simulink model "ahrs_wrk"  (R2021b)
settings: Solver=ode1be  StartTime=0.0  StopTime=tsc.Time(end)  FixedStep=0.01  RelTol=1e-3
values from neighbouring files (symbols this model uses):
  tsc = flatball_6dof_post( simout.logsout, disc, amb)    [flatball_6dof_wrk.m]    (also in hummel_thesis_mdl_validation.m = flatball_6dof_post( logsout, disc, amb))
libraries: mspfiltlib x1
settings Model: Creator=schae  LastModifiedBy=schae

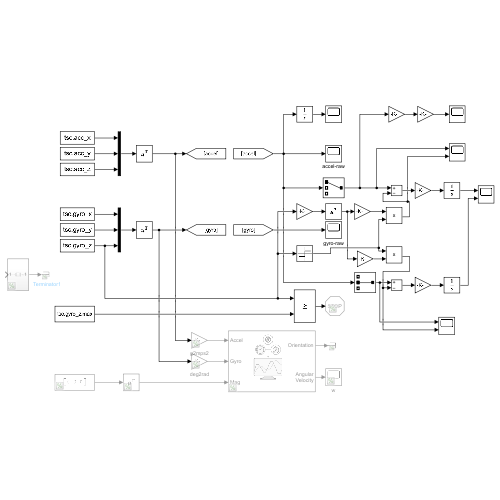
[thumbnail: Simulink's stored preview of the top-level diagram]
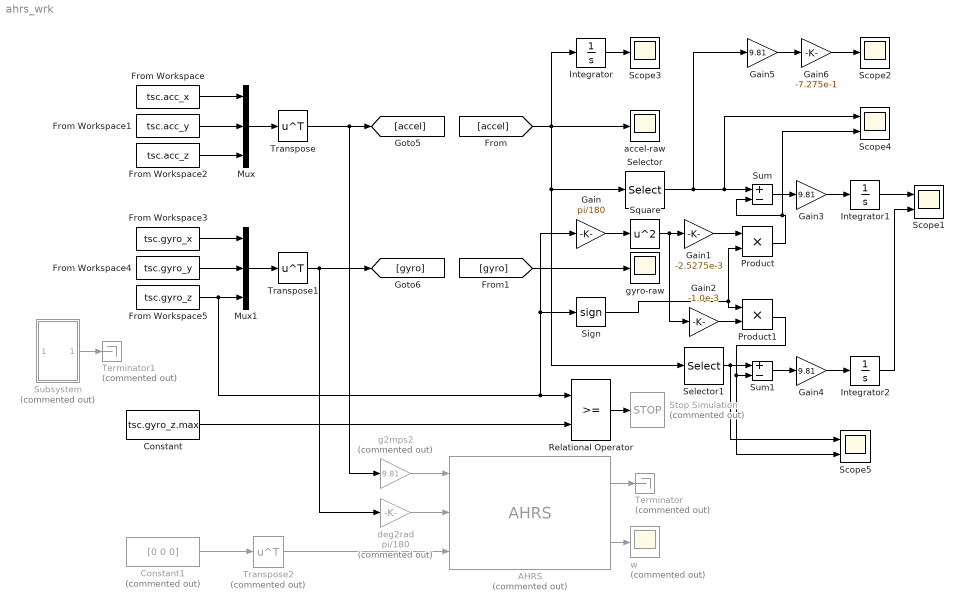
== system ahrs_wrk ==
  AHRS : mspfiltlib/AHRS  Commented=on  DispRefFrame=ENU  DecimationFactor=1  InitialProcessNoise=ahrsfilter.defaultProcessNoise  OrientationFormat=Rotation matrix  SimulateUsing=Interpreted execution  AccelerometerNoise=0.0001924722  GyroscopeNoise=9.1385e-5  MagnetometerNoise=0.1  GyroscopeDriftNoise=3.0462e-13  LinearAccelerationNoise=0.0096236100000000012  MagneticDisturbanceNoise=0.5  LinearAccelerationDecayFactor=0.5  MagneticDisturbanceDecayFactor=0.5  ExpectedMagneticFieldStrength=50
      settings: SourceProductBaseCode=TF,NV
  Constant : Constant  Value=tsc.gyro_z.max
  Constant1 : Constant  Commented=on  Value=[0 0 0]
  From Workspace : FromWorkspace  VariableName=tsc.acc_x  SampleTime=0.01  OutputAfterFinalValue=Holding final value
  From Workspace1 : FromWorkspace  VariableName=tsc.acc_y  SampleTime=0.01  OutputAfterFinalValue=Holding final value
  From Workspace2 : FromWorkspace  VariableName=tsc.acc_z  SampleTime=0.01  OutputAfterFinalValue=Holding final value
  From Workspace3 : FromWorkspace  VariableName=tsc.gyro_x  SampleTime=0.01  OutputAfterFinalValue=Holding final value
  From Workspace4 : FromWorkspace  VariableName=tsc.gyro_y  SampleTime=0.01  OutputAfterFinalValue=Holding final value
  From Workspace5 : FromWorkspace  VariableName=tsc.gyro_z  SampleTime=0.01  OutputAfterFinalValue=Holding final value
  Gain : Gain  Gain=pi/180
  Gain1 : Gain  Gain=-2.5275e-3
  Gain2 : Gain  Gain=-1.0e-3
  Gain3 : Gain  Gain=9.81
  Gain4 : Gain  Gain=9.81
  Gain5 : Gain  Gain=9.81
  Gain6 : Gain  Gain=-7.275e-1
  Integrator : Integrator
  Integrator1 : Integrator
  Integrator2 : Integrator
  Mux : Mux  Inputs=3
  Mux1 : Mux  Inputs=3
  Product : Product
  Product1 : Product
  Relational Operator : RelationalOperator  OutDataTypeStr=boolean  RndMeth=Simplest
  Scope1 : Scope  NumInputPorts=2
  Scope2 : Scope
  Scope3 : Scope
  Scope4 : Scope  NumInputPorts=2
  Scope5 : Scope  NumInputPorts=2
  Selector : Selector  InputPortWidth=3  IndexOptions=Index vector (dialog)  Indices=[1]  OutputSizes=1
  Selector1 : Selector  InputPortWidth=3  IndexOptions=Index vector (dialog)  Indices=[2]  OutputSizes=1
  Sign : Signum
  Square : Math  Operator=square  SaturateOnIntegerOverflow=on
  Stop Simulation : Stop  Commented=on
  Subsystem : Subsystem  Commented=on
  Sum : Sum  Inputs=+-
  Sum1 : Sum  Inputs=+-
  Terminator : Terminator  Commented=on
  Terminator1 : Terminator  Commented=on
  Transpose : Math  Operator=transpose  SaturateOnIntegerOverflow=on
  Transpose1 : Math  Operator=transpose  SaturateOnIntegerOverflow=on
  Transpose2 : Math  Commented=on  Operator=transpose  SaturateOnIntegerOverflow=on
  accel-raw : Scope
  deg2rad : Gain  Commented=on  Gain=pi/180
  g2mps2 : Gain  Commented=on  Gain=9.81
  gyro-raw : Scope
  w : Scope  Commented=on
  wires:
  From Workspace2/1 -> Mux/3
  From Workspace1/1 -> Mux/2
  From Workspace3/1 -> Mux1/1
  Mux/1 -> Transpose/1
  From Workspace/1 -> Mux/1
  From Workspace5/1 -> Sign/1, Gain/1, Relational Operator/1, Mux1/3
  Mux1/1 -> Transpose1/1
  From Workspace4/1 -> Mux1/2
  [gyro] -> gyro-raw/1
  Integrator/1 -> Scope3/1
  Constant/1 -> Relational Operator/2
  Relational Operator/1 -> Stop Simulation/1
  Constant1/1 -> Transpose2/1
  AHRS/2 -> w/1
  Transpose/1 -> g2mps2/1, [accel]
  Transpose1/1 -> deg2rad/1, [gyro]
  Transpose2/1 -> AHRS/3
  g2mps2/1 -> AHRS/1
  deg2rad/1 -> AHRS/2
  AHRS/1 -> Terminator/1
  Subsystem/1(Out1) -> Terminator1/1
  Selector/1 -> Gain5/1, Scope4/1, Sum/1
  Gain/1 -> Square/1
  Square/1 -> Gain2/1, Gain1/1
  Selector1/1 -> Sum1/1, Scope5/1
  Integrator1/1 -> Scope1/1
  Sum/1 -> Gain3/1
  Sum1/1 -> Gain4/1
  Integrator2/1 -> Scope1/2
  [accel] -> Selector/1, Selector1/1, Integrator/1, accel-raw/1
  Gain3/1 -> Integrator1/1
  Gain4/1 -> Integrator2/1
  Gain5/1 -> Gain6/1
  Gain6/1 -> Scope2/1
  Gain1/1 -> Product/1
  Sign/1 -> Product1/1, Product/2
  Product/1 -> Scope4/2, Sum/2
  Gain2/1 -> Product1/2
  Product1/1 -> Scope5/2, Sum1/2

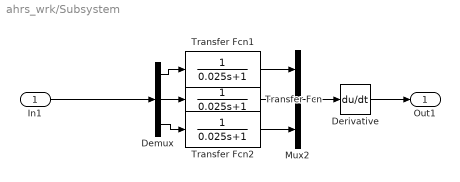
== system ahrs_wrk/Subsystem ==
  In1 : Inport
  Demux : Demux  Outputs=3
  Derivative : Derivative
  Mux2 : Mux  Inputs=3
  Transfer Fcn : TransferFcn  Denominator=[0.025 1]
  Transfer Fcn1 : TransferFcn  Denominator=[0.025 1]
  Transfer Fcn2 : TransferFcn  Denominator=[0.025 1]
  Out1 : Outport
  wires:
  Transfer Fcn/1 -> Mux2/2
  Demux/1 -> Transfer Fcn1/1
  Mux2/1 -> Derivative/1
  Demux/2 -> Transfer Fcn/1
  Transfer Fcn1/1 -> Mux2/1
  Transfer Fcn2/1 -> Mux2/3
  Demux/3 -> Transfer Fcn2/1
  In1/1 -> Demux/1
  Derivative/1 -> Out1/1
